simulink model "form_control"  (R2021a)
settings: Solver=VariableStepAuto  StartTime=0.0  StopTime=10.0  RelTol=1e-3
values from neighbouring files (symbols this model uses):
  altitude_d = 5    [run_swarm.m]
  altitude_i = 0    [run_swarm.m]
  b = fir1(filter_order, cutoff_frequency)    [lowpassfilter.m]    (also in run_swarm.m = 1.14e-07)
  g = 9.81    [run_swarm.m]
  I_xx = 4.856e-3    (= 0.004856)    [run_swarm.m]
  I_yy = 4.856e-3    (= 0.004856)    [run_swarm.m]
  I_zz = 8.801e-3    (= 0.008801)    [run_swarm.m]
  Im = 3.357e-5    (= 3.357e-05)    [run_swarm.m]
  k = 2.980e-6    (= 2.98e-06)    [run_swarm.m]
  l = legend(' Leader Position', ' Follower 1 Position','Follower 2 Position','Follower 3 Position')    [Untitled2.m]    (also in run_formation.m; run_swarm.m = legend('$\phi$ Current Y ', '$\phi_d$ Desired Y'); trajVis.m = legend('Desired Trajectory','Actual Trajectory'))
  m = 2    [master_control.m]    (also in run_swarm.m = 0.468)
  pitch_d = -0.1    [run_swarm.m]
  pitch_i = 0    [run_swarm.m]
  roll_d = 0.1    [run_swarm.m]
  roll_i = 0    [run_swarm.m]
  x_i = 0    [run_swarm.m]
  y_i = 0    [run_swarm.m]
  yaw_d = 0.3    [run_swarm.m]
  yaw_i = 0    [run_swarm.m]
libraries: slpidlib x4
settings Model: Creator=templ  LastModifiedBy=templ
settings SolverCC: ZeroCrossAlgorithm=Adaptive
settings DataIOCC: ReturnWorkspaceOutputs=off
settings DebuggingCC: IgnoredZcDiagnostic=none

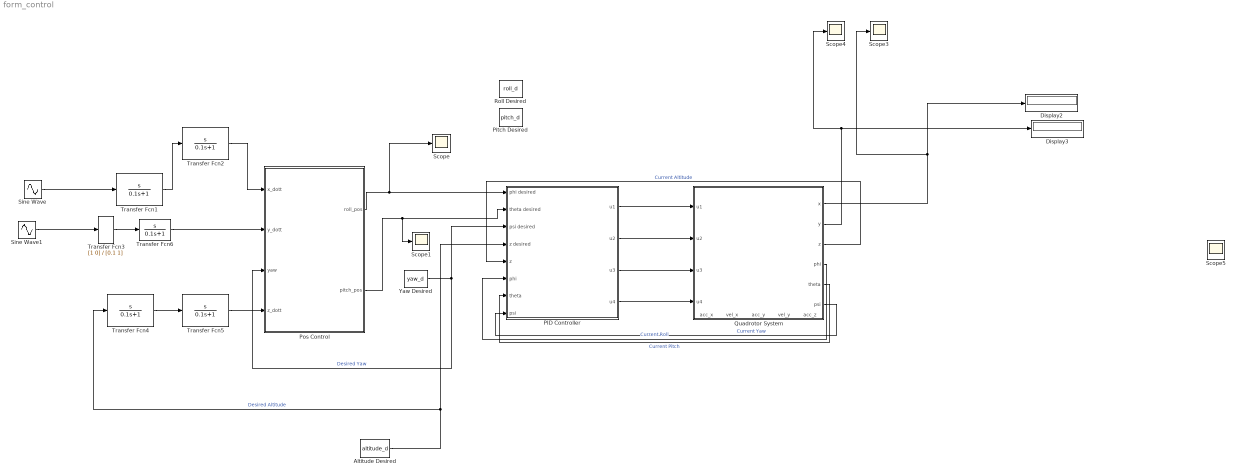
== system form_control ==
  Altitude Desired : Constant  Value=altitude_d
  Display2 : Display
  Display3 : Display
  PID Controller : Subsystem
  Pitch Desired : Constant  Value=pitch_d
  Pos Control : Subsystem
  Quadrotor System : Subsystem
      settings: PortSchema="{\"entries\":[{\"content\":{\"sides\":[{\"content\":{\"connectorIds\":[\"In1\",\"In2\",\"In3\",\"In4\"]},\"type\":\"ConnectorPlacement.EquallySpacedRectSide\",\"uuid\":\"996ed3cc-9aaf-410e-b93a-635ba5fc3cd9\"},{\"content\":{\"connectorIds\":[\"Out1\",\"Out2\",\"Out3\",\"Out4\",\"Out5\",\"Out6\"],\"side\":\"RIGHT\"},\"type\":\"ConnectorPlacement.EquallySpacedRectSide\",\"uuid\":\"7f76db3a-2ef6-433f-bd76-6f00d3bb4716\"},{\"content\":{\"connectorIds\":[],\"side\":\"TOP\"},\"type\":\"ConnectorPlacement.EquallySpacedRectSide\",\"uuid\":\"aa5fab1b-1d66-4c7a-823f-11c675c2f3d7\"},{\"content\":{\"connectorIds\":[\"Out7\",\"Out8\",\"Out9\",\"Out10\",\"Out11\"],\"side\":\"BOTTOM\"},\"type\":\"ConnectorPlacement.EquallySpacedRectSide\",\"uuid\":\"3e671b71-6d8e-4eea-a1dc-38ca984631fc\"}]},\"type\":\"ConnectorPlacement.EquallySpacedConnector\",\"uuid\":\"affe78d5-0f1f-4e1a-8cab-0d93ed3cb974\"}],\"packageUris\":[\"http://schema.mathworks.com/mf0/Connector/R2020b\"],\"version\":\"1.0\"}"
      mask Display: image('C:\Users\angel\OneDrive - Universidad Politécnica de Yucatán\CIMAT\1st semester\Robotic Systems Modeling and Control\Project\Quadrotor\images\quadrotor.jpg');
  Roll Desired : Constant  Value=roll_d
  Scope{,1,3..5} (5 alike) : Scope
  Sine Wave : Sin  SampleTime=0
  Sine Wave1 : Sin  SampleTime=0
  Transfer Fcn{1..6} (6 alike) : TransferFcn  Numerator=[1 0]  Denominator=[0.1 1]
  Yaw Desired : Constant  Value=yaw_d
  wires:
  Quadrotor System/1(x) -> Scope3/1, Display2/1
  Quadrotor System/3(z) -> PID Controller/5(z)  "Current Altitude"
  Quadrotor System/2(y) -> Scope4/1, Display3/1
  Quadrotor System/5(theta) -> PID Controller/7(theta)  "Current Pitch"
  Quadrotor System/4(phi) -> PID Controller/6(phi)  "Current Roll"
  Altitude Desired/1 -> Transfer Fcn4/1, PID Controller/4(z desired)  "Desired Altitude"
  Yaw Desired/1 -> PID Controller/3(psi desired), Pos Control/3(yaw)  "Desired Yaw"
  PID Controller/3(u3) -> Quadrotor System/3(u3)
  PID Controller/4(u4) -> Quadrotor System/4(u4)
  PID Controller/2(u2) -> Quadrotor System/2(u2)
  Quadrotor System/6(psi) -> PID Controller/8(psi)  "Current Yaw"
  PID Controller/1(u1) -> Quadrotor System/1(u1)
  Transfer Fcn2/1 -> Pos Control/1(x_dott)
  Sine Wave/1 -> Transfer Fcn1/1
  Sine Wave1/1 -> Transfer Fcn3/1
  Transfer Fcn6/1 -> Pos Control/2(y_dott)
  Pos Control/1(roll_pos) -> Scope/1, PID Controller/1(phi desired)
  Pos Control/2(pitch_pos) -> Scope1/1, PID Controller/2(theta desired)
  Transfer Fcn5/1 -> Pos Control/4(z_dott)
  Transfer Fcn4/1 -> Transfer Fcn5/1
  Transfer Fcn1/1 -> Transfer Fcn2/1
  Transfer Fcn3/1 -> Transfer Fcn6/1

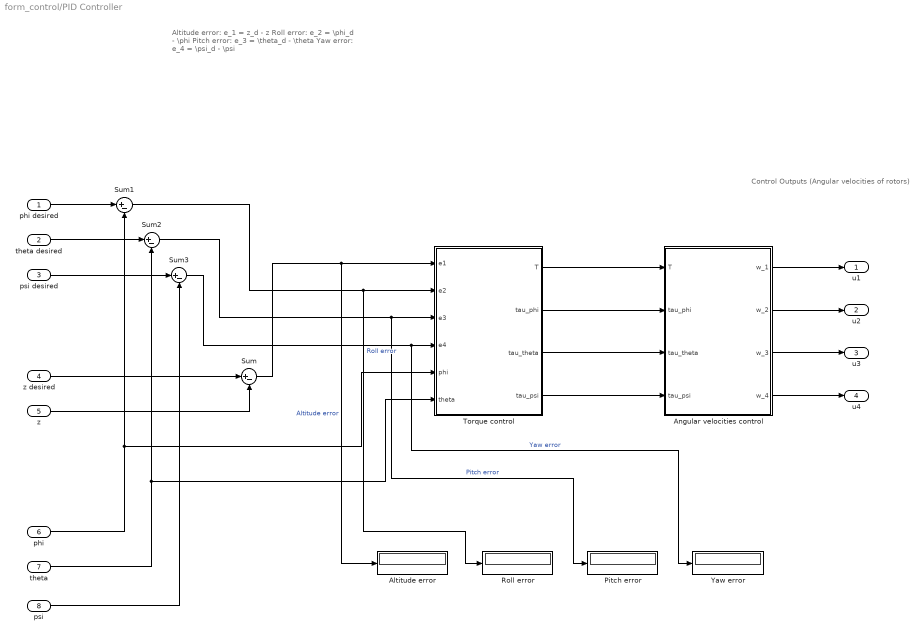
== system form_control/PID Controller ==
  note: Control Outputs
      | (Angular velocities of rotors)
  note: Altitude error: e_1 = z_d - z
      | Roll error: e_2 = \phi_d - \phi
      | Pitch error: e_3 = \theta_d - \theta
      | Yaw error: e_4 = \psi_d - \psi
  phi desired : Inport
  theta desired : Inport  Port=2
  psi desired : Inport  Port=3
  z desired : Inport  Port=4
  z : Inport  Port=5
  phi : Inport  Port=6
  theta : Inport  Port=7
  psi : Inport  Port=8
  Altitude error : Display
  Angular velocities control : Subsystem
  Pitch error : Display
  Roll error : Display
  Sum{,1..3} (4 alike) : Sum  Inputs=|+-
  Torque control : Subsystem
  Yaw error : Display
  u1 : Outport
  u2 : Outport  Port=2
  u3 : Outport  Port=3
  u4 : Outport  Port=4
  wires:
  z desired/1 -> Sum/1
  z/1 -> Sum/2
  Sum/1 -> Altitude error/1, Torque control/1(e1)  "Altitude error"
  phi desired/1 -> Sum1/1
  phi/1 -> Torque control/5("phi "), Sum1/2
  theta desired/1 -> Sum2/1
  theta/1 -> Sum2/2, Torque control/6("theta ")
  psi desired/1 -> Sum3/1
  psi/1 -> Sum3/2
  Sum1/1 -> Roll error/1, Torque control/2(e2)  "Roll error"
  Sum2/1 -> Pitch error/1, Torque control/3(e3)  "Pitch error"
  Sum3/1 -> Yaw error/1, Torque control/4(e4)  "Yaw error"
  Torque control/1(T) -> Angular velocities control/1(T)
  Torque control/2(tau_phi) -> Angular velocities control/2(tau_phi)
  Torque control/3(tau_theta) -> Angular velocities control/3(tau_theta)
  Torque control/4(tau_psi) -> Angular velocities control/4("tau_psi ")
  Angular velocities control/1(w_1) -> u1/1
  Angular velocities control/2(w_2) -> u2/1
  Angular velocities control/3(w_3) -> u3/1
  Angular velocities control/4("w_4 ") -> u4/1

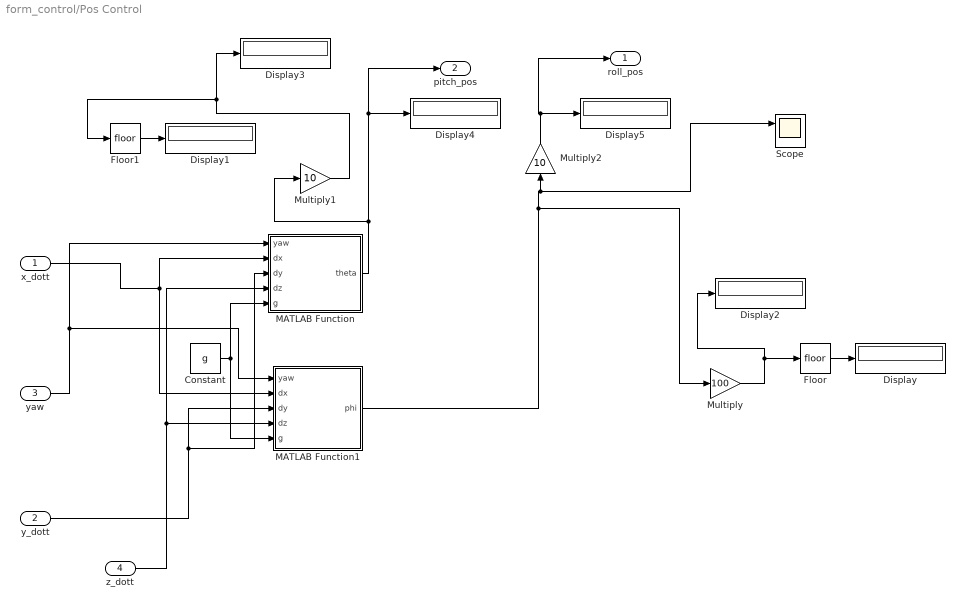
== system form_control/Pos Control ==
  x_dott : Inport
  y_dott : Inport  Port=2
  yaw : Inport  Port=3
  z_dott : Inport  Port=4
  Constant : Constant  Value=g
  Display{,1..5} (6 alike) : Display
  Floor : Rounding
  Floor1 : Rounding
  MATLAB Function : MATLAB Function  TreatAsAtomicUnit=on
  MATLAB Function1 : MATLAB Function  TreatAsAtomicUnit=on
  Multiply : Gain  Gain=100
  Multiply1 : Gain  Gain=10
  Multiply2 : Gain  Gain=10
  Scope : Scope  NumInputPorts=2
  roll_pos : Outport
  pitch_pos : Outport  Port=2
  wires:
  yaw/1 -> MATLAB Function/1(yaw), MATLAB Function1/1(yaw)
  Constant/1 -> MATLAB Function/5(g), MATLAB Function1/5(g)
  MATLAB Function1/1(phi) -> Multiply2/1, Scope/1, Multiply/1
  x_dott/1 -> MATLAB Function1/2(dx), MATLAB Function/2(dx)
  y_dott/1 -> MATLAB Function/3(dy), MATLAB Function1/3(dy)
  Multiply/1 -> Display2/1, Floor/1
  z_dott/1 -> MATLAB Function1/4(dz), MATLAB Function/4(dz)
  MATLAB Function/1(theta) -> pitch_pos/1, Display4/1, Multiply1/1
  Floor/1 -> Display/1
  Multiply1/1 -> Display3/1, Floor1/1
  Floor1/1 -> Display1/1
  Multiply2/1 -> roll_pos/1, Display5/1

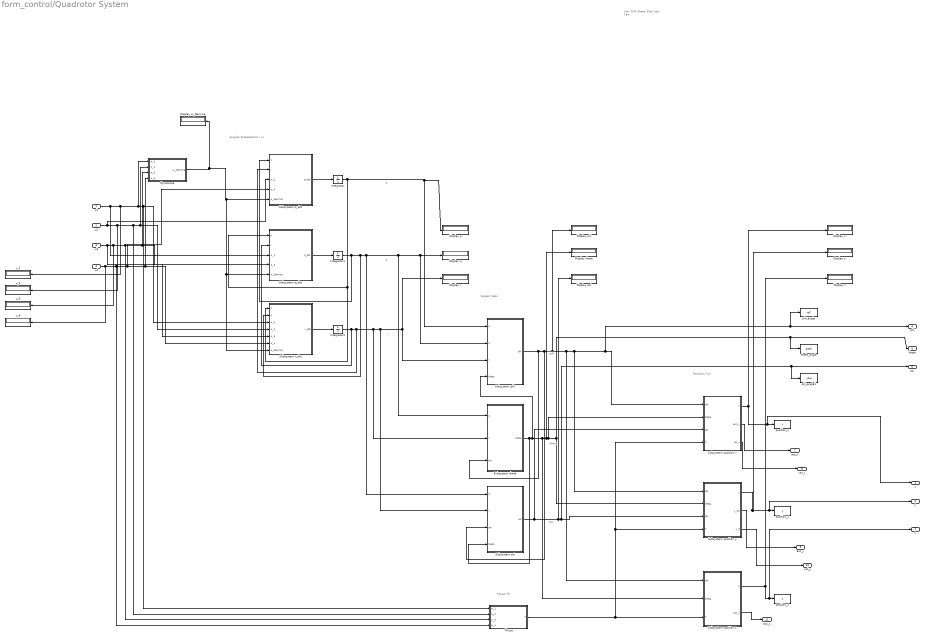
== system form_control/Quadrotor System ==
  note: Angular Accelerations (\nu)
  note: .
  note: \phi: Roll
      | \theta: Pitch
      | \psi: Yaw
  note: Positions (\xi)
  note: Angles (\eta)
  note: Thrust (T)
  note: p
  note: q
  note: r
  note: \phi
  note: \theta
  note: \psi
  u1 : Inport
  u2 : Inport  Port=2
  u3 : Inport  Port=3
  u4 : Inport  Port=4
  Display p : Display
  Display phi : Display
  Display psi : Display
  Display q : Display
  Display r : Display
  Display theta : Display
  Display w_Gamma : Display
  Display x : Display
  Display y : Display
  Display z : Display
  Gyroscope : MATLAB Function  TreatAsAtomicUnit=on
  Integrator : Integrator
  Integrator1 : Integrator
  Integrator2 : Integrator
  Subsystem p_dot : Subsystem
  Subsystem phi : Subsystem
  Subsystem position x : Subsystem
  Subsystem position y : Subsystem
  Subsystem position z : Subsystem
  Subsystem psi : Subsystem
  Subsystem q_dot : Subsystem
  Subsystem r_dot : Subsystem
  Subsystem theta : Subsystem
  Thrust : MATLAB Function  TreatAsAtomicUnit=on
  phi_angle : ToWorkspace  VariableName=roll  SampleTime=-1
  phi_angle1 : ToWorkspace  VariableName=yaw  SampleTime=-1
  position_x : ToWorkspace  VariableName=x  SampleTime=-1
  position_y : ToWorkspace  VariableName=y  SampleTime=-1
  position_z : ToWorkspace  VariableName=z  SampleTime=-1
  theta_angle : ToWorkspace  VariableName=pitch  SampleTime=-1
  u_{1..4} (4 alike) : Display
  x : Outport
  y : Outport  Port=2
  z : Outport  Port=3
  phi : Outport  Port=4
  theta : Outport  Port=5
  psi : Outport  Port=6
  acc_x : Outport  Port=7
  vel_x : Outport  Port=8
  acc_y : Outport  Port=9
  vel_y : Outport  Port=10
  acc_z : Outport  Port=11
  wires:
  u1/1 -> Subsystem q_dot/3(w_1), u_1/1, Gyroscope/1(w_1), Subsystem r_dot/3(w_1), Thrust/1(w_1)
  u2/1 -> Subsystem p_dot/3(w_2), u_2/1, Gyroscope/2(w_2), Subsystem r_dot/4(w_2), Thrust/2(w_2)
  u3/1 -> Subsystem q_dot/4(w_3), Gyroscope/3(w_3), Subsystem r_dot/5(w_3), Thrust/3(w_3), u_3/1
  u4/1 -> u_4/1, Gyroscope/4(w_4), Subsystem r_dot/6(w_4), Subsystem p_dot/4(w_4), Thrust/4(w_4)
  Thrust/1(T) -> Subsystem position y/4("T "), Subsystem position x/4(T), Subsystem position z/3(T)
  Subsystem phi/1("phi ") -> Subsystem theta/3("phi "), Subsystem psi/3(phi), Display phi/1, Subsystem position z/1("phi "), Subsystem position y/1("phi "), phi_angle/1, phi/1, Subsystem position x/1("phi ")
  Subsystem psi/1(psi) -> Subsystem position x/3("psi "), Display psi/1, phi_angle1/1, psi/1, Subsystem position y/3("psi ")
  Subsystem position x/1(x) -> x/1, position_x/1, Display x/1
  Subsystem position z/1(z) -> z/1, position_z/1, Display z/1
  Subsystem position y/1("y ") -> Display y/1, y/1, position_y/1
  Gyroscope/1(w_Gamma) -> Display w_Gamma/1, Subsystem r_dot/7(w_Gamma), Subsystem q_dot/5("w_Gamma "), Subsystem p_dot/5("w_Gamma ")
  Subsystem p_dot/1(p_dot) -> Integrator/1
  Subsystem q_dot/1(q_dot) -> Integrator1/1
  Subsystem r_dot/1(r_dot) -> Integrator2/1
  Integrator/1 -> Subsystem r_dot/1("p "), Subsystem q_dot/1("p "), Display p/1, Subsystem phi/1(p)
  Integrator2/1 -> Subsystem theta/2(r), Subsystem psi/2(r), Display r/1, Subsystem phi/3(r), Subsystem p_dot/2(r), Subsystem q_dot/2(r)
  Integrator1/1 -> Subsystem p_dot/1(q), Subsystem psi/1(q), Subsystem theta/1(q), Display q/1, Subsystem phi/2(q), Subsystem r_dot/2(q)
  Subsystem theta/1(theta) -> Subsystem psi/4(theta), Subsystem phi/4(theta), Subsystem position z/2("theta "), Display theta/1, Subsystem position x/2("theta "), theta_angle/1, theta/1, Subsystem position y/2("theta ")
  Subsystem position x/2(acc_x) -> acc_x/1
  Subsystem position x/3(vel_x) -> vel_x/1
  Subsystem position y/2(y_dd) -> acc_y/1
  Subsystem position y/3(y_d) -> vel_y/1
  Subsystem position z/2(acc_z) -> acc_z/1

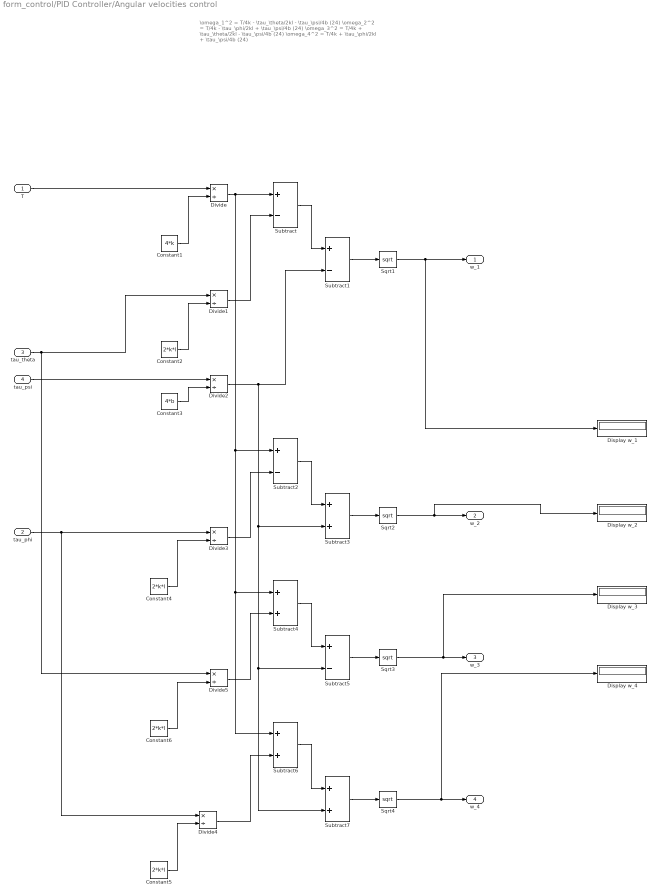
== system form_control/PID Controller/Angular velocities control ==
  note: \omega_1^2 = T/4k - \tau_\theta/2kl - \tau_\psi/4b   (24)
      |
      | \omega_2^2 = T/4k - \tau_\phi/2kl + \tau_\psi/4b   (24)
      |
      | \omega_3^2 = T/4k + \tau_\theta/2kl - \tau_\psi/4b   (24)
      |
      | \omega_4^2 = T/4k + \tau_\phi/2kl + \tau_\psi/4b   (24)
  T : Inport
  tau_phi : Inport  Port=2
  tau_theta : Inport  Port=3
  "tau_psi " : Inport  Port=4
  Constant1 : Constant  Value=4*k
  Constant{2,4..6} (4 alike) : Constant  Value=2*k*l
  Constant3 : Constant  Value=4*b
  Display w_{1..4} (4 alike) : Display
  Divide{,1..5} (6 alike) : Product  Inputs=*/
  Sqrt{1..4} (4 alike) : Sqrt  OutputSignalType=real  SaturateOnIntegerOverflow=on
  Subtract{,1..2,5} (4 alike) : Sum  Inputs=+-
  Subtract{3..4,6..7} (4 alike) : Sum
  w_1 : Outport
  w_2 : Outport  Port=2
  w_3 : Outport  Port=3
  "w_4 " : Outport  Port=4
  wires:
  Constant1/1 -> Divide/2
  T/1 -> Divide/1
  Divide/1 -> Subtract4/1, Subtract6/1, Subtract2/1, Subtract/1
  Constant2/1 -> Divide1/2
  tau_theta/1 -> Divide5/1, Divide1/1
  Divide1/1 -> Subtract/2
  Subtract/1 -> Subtract1/1
  Constant3/1 -> Divide2/2
  Subtract1/1 -> Sqrt1/1
  Sqrt1/1 -> Display w_1/1, w_1/1
  Constant4/1 -> Divide3/2
  tau_phi/1 -> Divide4/1, Divide3/1
  Divide3/1 -> Subtract2/2
  Subtract2/1 -> Subtract3/1
  "tau_psi "/1 -> Divide2/1
  Divide2/1 -> Subtract7/2, Subtract5/2, Subtract3/2, Subtract1/2
  Sqrt2/1 -> Display w_2/1, w_2/1
  Subtract3/1 -> Sqrt2/1
  Constant6/1 -> Divide5/2
  Divide5/1 -> Subtract4/2
  Subtract5/1 -> Sqrt3/1
  Subtract4/1 -> Subtract5/1
  Sqrt3/1 -> Display w_3/1, w_3/1
  Subtract7/1 -> Sqrt4/1
  Constant5/1 -> Divide4/2
  Divide4/1 -> Subtract6/2
  Subtract6/1 -> Subtract7/1
  Sqrt4/1 -> Display w_4/1, "w_4 "/1

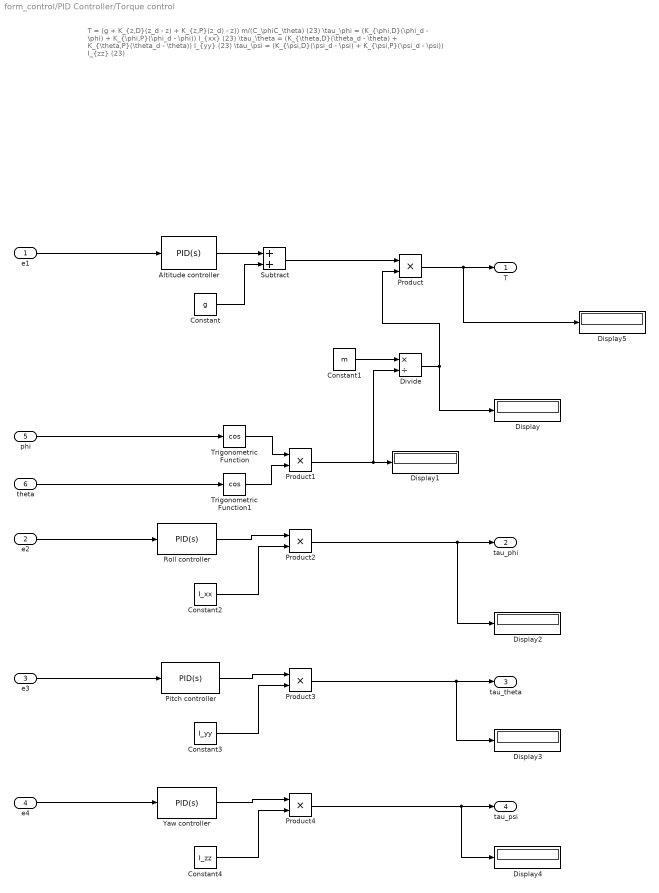
== system form_control/PID Controller/Torque control ==
  note: T = (g + K_{z,D}(z_d - z) + K_{z,P}(z_d) - z)) m/(C_\phiC_\theta)     (23)
      |
      | \tau_\phi = (K_{\phi,D}(\phi_d - \phi) + K_{\phi,P}(\phi_d - \phi)) I_{xx}                   (23)
      |
      | \tau_\theta = (K_{\theta,D}(\theta_d - \theta) + K_{\theta,P}(\theta_d - \theta)) I_{yy}                    (23)
      |
      | \tau_\psi = (K_{\psi,D}(\psi_d - \psi) + K_{\psi,P}(\psi_d - \psi)) I_{zz}                (23)
  e1 : Inport
  e2 : Inport  Port=2
  e3 : Inport  Port=3
  e4 : Inport  Port=4
  "phi " : Inport  Port=5
  "theta " : Inport  Port=6
  Altitude controller : slpidlib/PID Controller  Controller=PID  Form=Parallel  TimeDomain=Continuous-time  UseExternalTs=off  SampleTime=-1  IntegratorMethod=Forward Euler  FilterMethod=Forward Euler  ControllerParametersSource=internal  P=57  I=0.001  D=23  UseFilter=on  N=572.770791824146  TunerSelectOption=Transfer Function Based (PID Tuner App)  InitialConditionSource=internal  InitialConditionForIntegrator=0  InitialConditionForFilter=0  DifferentiatorICPrevScaledInput=0  ExternalReset=none  TrackingMode=off  Kt=1  LimitOutput=on  SatLimitsSource=internal  UpperSaturationLimit=5  LowerSaturationLimit=-5  LinearizeAsGain=on  AntiWindupMode=none  Kb=1  POutMin=[]  POutMax=[]  IOutMin=[]  IOutMax=[]  DOutMin=[]  DOutMax=[]  NOutMin=[]  NOutMax=[]  SumOutMin=[]  SumOutMax=[]  SaturationOutMin=[]  SaturationOutMax=[]  PParamMin=[]  PParamMax=[]  IParamMin=[]  IParamMax=[]  DParamMin=[]  DParamMax=[]  NParamMin=[]  NParamMax=[]  KbParamMin=[]  KbParamMax=[]  KtParamMin=[]  KtParamMax=[]  KbOutMin=[]  KbOutMax=[]  KtOutMin=[]  KtOutMax=[]  IntegratorOutMin=[]  IntegratorOutMax=[]  FilterOutMin=[]  FilterOutMax=[]  SumI1OutMin=[]  SumI1OutMax=[]  SumI2OutMin=[]  SumI2OutMax=[]  SumI3OutMin=[]  SumI3OutMax=[]  SumI4OutMin=[]  SumI4OutMax=[]  SumDOutMin=[]  SumDOutMax=[]  DifferentiatorOutMin=[]  DifferentiatorOutMax=[]  FilterDiffOutCoefMin=[]  FilterDiffOutCoefMax=[]  ReciprocalOutMin=[]  ReciprocalOutMax=[]  SumDenOutMin=[]  SumDenOutMax=[]  SumNumOutMin=[]  SumNumOutMax=[]  DivideOutMin=[]  DivideOutMax=[]  UdiffTsProdOutMin=[]  UdiffTsProdOutMax=[]  NTsProdOutMin=[]  NTsProdOutMax=[]  UintegralTsProdOutMin=[]  UintegralTsProdOutMax=[]  UngainTsProdOutMin=[]  UngainTsProdOutMax=[]  IntegratorContinuousStateAttributes=''  IntegratorStateMustResolveToSignalObject=off  IntegratorRTWStateStorageClass=Auto  FilterContinuousStateAttributes=''  FilterStateMustResolveToSignalObject=off  FilterRTWStateStorageClass=Auto  ParallelPVariant=InternalParameters  IdealPVariant=Disabled  IVariant=InternalParameters  DVariant=InternalParameters  IntegratorVariant=Continuous  SatVariant=Enabled  AWVariant=Passthrough  PCopyVariant=Disabled  TRVariant=Disabled  FdbkBlocksVariant=Forward  IdealPFdbkVariant=Disabled  SatFdbkVariant=Disabled  DerivativeFilterVariant=ContFilter  NVariant=InternalParameters  NCopyVariant=Disabled  FilterICVariant=InternalICsFilter  IntegratorICVariant=InternalICs  ExternalResetVariant=Disabled  TRSumVariant=Passthrough  SumFdbkVariant=Disabled  SumVariant=Sum_PID  TsampFilterVariant=InternalTs  TsampNgainVariant=Passthrough  TsampIntegralVariant=Passthrough  ExternalSaturationOutDataTypeStr=Inherit: Same as second input
  Constant : Constant  Value=g
  Constant1 : Constant  Value=m
  Constant2 : Constant  Value=I_xx
  Constant3 : Constant  Value=I_yy
  Constant4 : Constant  Value=I_zz
  Display{,1..5} (6 alike) : Display
  Divide : Product  Inputs=*/
  Pitch controller : slpidlib/PID Controller  Controller=PID  Form=Parallel  TimeDomain=Continuous-time  UseExternalTs=off  SampleTime=-1  IntegratorMethod=Forward Euler  FilterMethod=Forward Euler  ControllerParametersSource=internal  P=55  I=0.01  D=11  UseFilter=on  N=1414.64809761679  TunerSelectOption=Transfer Function Based (PID Tuner App)  InitialConditionSource=internal  InitialConditionForIntegrator=0  InitialConditionForFilter=0  DifferentiatorICPrevScaledInput=0  ExternalReset=none  TrackingMode=off  Kt=1  LimitOutput=on  SatLimitsSource=internal  UpperSaturationLimit=0.9  LowerSaturationLimit=-0.9  LinearizeAsGain=on  AntiWindupMode=none  Kb=1  POutMin=[]  POutMax=[]  IOutMin=[]  IOutMax=[]  DOutMin=[]  DOutMax=[]  NOutMin=[]  NOutMax=[]  SumOutMin=[]  SumOutMax=[]  SaturationOutMin=[]  SaturationOutMax=[]  PParamMin=[]  PParamMax=[]  IParamMin=[]  IParamMax=[]  DParamMin=[]  DParamMax=[]  NParamMin=[]  NParamMax=[]  KbParamMin=[]  KbParamMax=[]  KtParamMin=[]  KtParamMax=[]  KbOutMin=[]  KbOutMax=[]  KtOutMin=[]  KtOutMax=[]  IntegratorOutMin=[]  IntegratorOutMax=[]  FilterOutMin=[]  FilterOutMax=[]  SumI1OutMin=[]  SumI1OutMax=[]  SumI2OutMin=[]  SumI2OutMax=[]  SumI3OutMin=[]  SumI3OutMax=[]  SumI4OutMin=[]  SumI4OutMax=[]  SumDOutMin=[]  SumDOutMax=[]  DifferentiatorOutMin=[]  DifferentiatorOutMax=[]  FilterDiffOutCoefMin=[]  FilterDiffOutCoefMax=[]  ReciprocalOutMin=[]  ReciprocalOutMax=[]  SumDenOutMin=[]  SumDenOutMax=[]  SumNumOutMin=[]  SumNumOutMax=[]  DivideOutMin=[]  DivideOutMax=[]  UdiffTsProdOutMin=[]  UdiffTsProdOutMax=[]  NTsProdOutMin=[]  NTsProdOutMax=[]  UintegralTsProdOutMin=[]  UintegralTsProdOutMax=[]  UngainTsProdOutMin=[]  UngainTsProdOutMax=[]  IntegratorContinuousStateAttributes=''  IntegratorStateMustResolveToSignalObject=off  IntegratorRTWStateStorageClass=Auto  FilterContinuousStateAttributes=''  FilterStateMustResolveToSignalObject=off  FilterRTWStateStorageClass=Auto  ParallelPVariant=InternalParameters  IdealPVariant=Disabled  IVariant=InternalParameters  DVariant=InternalParameters  IntegratorVariant=Continuous  SatVariant=Enabled  AWVariant=Passthrough  PCopyVariant=Disabled  TRVariant=Disabled  FdbkBlocksVariant=Forward  IdealPFdbkVariant=Disabled  SatFdbkVariant=Disabled  DerivativeFilterVariant=ContFilter  NVariant=InternalParameters  NCopyVariant=Disabled  FilterICVariant=InternalICsFilter  IntegratorICVariant=InternalICs  ExternalResetVariant=Disabled  TRSumVariant=Passthrough  SumFdbkVariant=Disabled  SumVariant=Sum_PID  TsampFilterVariant=InternalTs  TsampNgainVariant=Passthrough  TsampIntegralVariant=Passthrough  ExternalSaturationOutDataTypeStr=Inherit: Same as second input
  Product{,1..4} (5 alike) : Product
  Roll controller : slpidlib/PID Controller  Controller=PID  Form=Parallel  TimeDomain=Continuous-time  UseExternalTs=off  SampleTime=-1  IntegratorMethod=Forward Euler  FilterMethod=Forward Euler  ControllerParametersSource=internal  P=55  I=0.01  D=18  UseFilter=on  N=1414.64809761679  TunerSelectOption=Transfer Function Based (PID Tuner App)  InitialConditionSource=internal  InitialConditionForIntegrator=0  InitialConditionForFilter=0  DifferentiatorICPrevScaledInput=0  ExternalReset=none  TrackingMode=off  Kt=1  LimitOutput=on  SatLimitsSource=internal  UpperSaturationLimit=0.9  LowerSaturationLimit=-0.9  LinearizeAsGain=on  AntiWindupMode=none  Kb=1  POutMin=[]  POutMax=[]  IOutMin=[]  IOutMax=[]  DOutMin=[]  DOutMax=[]  NOutMin=[]  NOutMax=[]  SumOutMin=[]  SumOutMax=[]  SaturationOutMin=[]  SaturationOutMax=[]  PParamMin=[]  PParamMax=[]  IParamMin=[]  IParamMax=[]  DParamMin=[]  DParamMax=[]  NParamMin=[]  NParamMax=[]  KbParamMin=[]  KbParamMax=[]  KtParamMin=[]  KtParamMax=[]  KbOutMin=[]  KbOutMax=[]  KtOutMin=[]  KtOutMax=[]  IntegratorOutMin=[]  IntegratorOutMax=[]  FilterOutMin=[]  FilterOutMax=[]  SumI1OutMin=[]  SumI1OutMax=[]  SumI2OutMin=[]  SumI2OutMax=[]  SumI3OutMin=[]  SumI3OutMax=[]  SumI4OutMin=[]  SumI4OutMax=[]  SumDOutMin=[]  SumDOutMax=[]  DifferentiatorOutMin=[]  DifferentiatorOutMax=[]  FilterDiffOutCoefMin=[]  FilterDiffOutCoefMax=[]  ReciprocalOutMin=[]  ReciprocalOutMax=[]  SumDenOutMin=[]  SumDenOutMax=[]  SumNumOutMin=[]  SumNumOutMax=[]  DivideOutMin=[]  DivideOutMax=[]  UdiffTsProdOutMin=[]  UdiffTsProdOutMax=[]  NTsProdOutMin=[]  NTsProdOutMax=[]  UintegralTsProdOutMin=[]  UintegralTsProdOutMax=[]  UngainTsProdOutMin=[]  UngainTsProdOutMax=[]  IntegratorContinuousStateAttributes=''  IntegratorStateMustResolveToSignalObject=off  IntegratorRTWStateStorageClass=Auto  FilterContinuousStateAttributes=''  FilterStateMustResolveToSignalObject=off  FilterRTWStateStorageClass=Auto  ParallelPVariant=InternalParameters  IdealPVariant=Disabled  IVariant=InternalParameters  DVariant=InternalParameters  IntegratorVariant=Continuous  SatVariant=Enabled  AWVariant=Passthrough  PCopyVariant=Disabled  TRVariant=Disabled  FdbkBlocksVariant=Forward  IdealPFdbkVariant=Disabled  SatFdbkVariant=Disabled  DerivativeFilterVariant=ContFilter  NVariant=InternalParameters  NCopyVariant=Disabled  FilterICVariant=InternalICsFilter  IntegratorICVariant=InternalICs  ExternalResetVariant=Disabled  TRSumVariant=Passthrough  SumFdbkVariant=Disabled  SumVariant=Sum_PID  TsampFilterVariant=InternalTs  TsampNgainVariant=Passthrough  TsampIntegralVariant=Passthrough  ExternalSaturationOutDataTypeStr=Inherit: Same as second input
  Subtract : Sum
  Trigonometric Function : Trigonometry  Operator=cos
  Trigonometric Function1 : Trigonometry  Operator=cos
  Yaw controller : slpidlib/PID Controller  Controller=PID  Form=Parallel  TimeDomain=Continuous-time  UseExternalTs=off  SampleTime=-1  IntegratorMethod=Forward Euler  FilterMethod=Forward Euler  ControllerParametersSource=internal  P=53  I=0.04  D=26.2  UseFilter=on  N=95.667343116538  TunerSelectOption=Transfer Function Based (PID Tuner App)  InitialConditionSource=internal  InitialConditionForIntegrator=0  InitialConditionForFilter=0  DifferentiatorICPrevScaledInput=0  ExternalReset=none  TrackingMode=off  Kt=1  LimitOutput=on  SatLimitsSource=internal  UpperSaturationLimit=5  LowerSaturationLimit=-5  LinearizeAsGain=on  AntiWindupMode=none  Kb=1  POutMin=[]  POutMax=[]  IOutMin=[]  IOutMax=[]  DOutMin=[]  DOutMax=[]  NOutMin=[]  NOutMax=[]  SumOutMin=[]  SumOutMax=[]  SaturationOutMin=[]  SaturationOutMax=[]  PParamMin=[]  PParamMax=[]  IParamMin=[]  IParamMax=[]  DParamMin=[]  DParamMax=[]  NParamMin=[]  NParamMax=[]  KbParamMin=[]  KbParamMax=[]  KtParamMin=[]  KtParamMax=[]  KbOutMin=[]  KbOutMax=[]  KtOutMin=[]  KtOutMax=[]  IntegratorOutMin=[]  IntegratorOutMax=[]  FilterOutMin=[]  FilterOutMax=[]  SumI1OutMin=[]  SumI1OutMax=[]  SumI2OutMin=[]  SumI2OutMax=[]  SumI3OutMin=[]  SumI3OutMax=[]  SumI4OutMin=[]  SumI4OutMax=[]  SumDOutMin=[]  SumDOutMax=[]  DifferentiatorOutMin=[]  DifferentiatorOutMax=[]  FilterDiffOutCoefMin=[]  FilterDiffOutCoefMax=[]  ReciprocalOutMin=[]  ReciprocalOutMax=[]  SumDenOutMin=[]  SumDenOutMax=[]  SumNumOutMin=[]  SumNumOutMax=[]  DivideOutMin=[]  DivideOutMax=[]  UdiffTsProdOutMin=[]  UdiffTsProdOutMax=[]  NTsProdOutMin=[]  NTsProdOutMax=[]  UintegralTsProdOutMin=[]  UintegralTsProdOutMax=[]  UngainTsProdOutMin=[]  UngainTsProdOutMax=[]  IntegratorContinuousStateAttributes=''  IntegratorStateMustResolveToSignalObject=off  IntegratorRTWStateStorageClass=Auto  FilterContinuousStateAttributes=''  FilterStateMustResolveToSignalObject=off  FilterRTWStateStorageClass=Auto  ParallelPVariant=InternalParameters  IdealPVariant=Disabled  IVariant=InternalParameters  DVariant=InternalParameters  IntegratorVariant=Continuous  SatVariant=Enabled  AWVariant=Passthrough  PCopyVariant=Disabled  TRVariant=Disabled  FdbkBlocksVariant=Forward  IdealPFdbkVariant=Disabled  SatFdbkVariant=Disabled  DerivativeFilterVariant=ContFilter  NVariant=InternalParameters  NCopyVariant=Disabled  FilterICVariant=InternalICsFilter  IntegratorICVariant=InternalICs  ExternalResetVariant=Disabled  TRSumVariant=Passthrough  SumFdbkVariant=Disabled  SumVariant=Sum_PID  TsampFilterVariant=InternalTs  TsampNgainVariant=Passthrough  TsampIntegralVariant=Passthrough  ExternalSaturationOutDataTypeStr=Inherit: Same as second input
  T : Outport
  tau_phi : Outport  Port=2
  tau_theta : Outport  Port=3
  tau_psi : Outport  Port=4
  wires:
  Constant/1 -> Subtract/2
  e1/1 -> Altitude controller/1
  Altitude controller/1 -> Subtract/1
  Subtract/1 -> Product/1
  Constant1/1 -> Divide/1
  Divide/1 -> Product/2, Display/1
  "phi "/1 -> Trigonometric Function/1
  "theta "/1 -> Trigonometric Function1/1
  Trigonometric Function/1 -> Product1/1
  Trigonometric Function1/1 -> Product1/2
  Product1/1 -> Display1/1, Divide/2
  Product/1 -> Display5/1, T/1
  e2/1 -> Roll controller/1
  Roll controller/1 -> Product2/1
  Constant2/1 -> Product2/2
  Product2/1 -> Display2/1, tau_phi/1
  Constant3/1 -> Product3/2
  Pitch controller/1 -> Product3/1
  Constant4/1 -> Product4/2
  Yaw controller/1 -> Product4/1
  e4/1 -> Yaw controller/1
  e3/1 -> Pitch controller/1
  Product3/1 -> Display3/1, tau_theta/1
  Product4/1 -> Display4/1, tau_psi/1

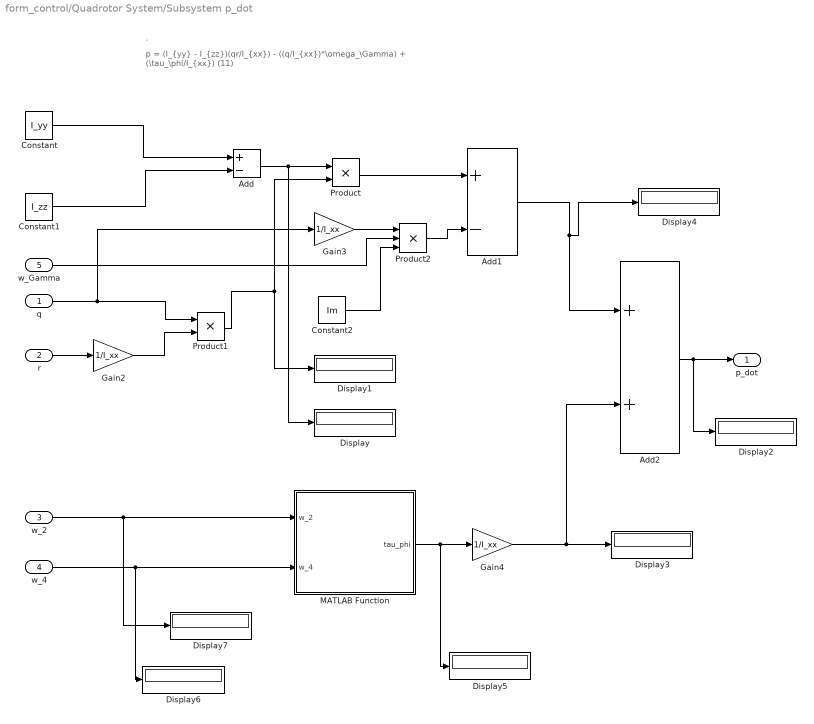
== system form_control/Quadrotor System/Subsystem p_dot ==
  note: p = (I_{yy} - I_{zz})(qr/I_{xx}) - ((q/I_{xx})*\omega_\Gamma) + (\tau_\phi/I_{xx}) (11)
  note: .
  q : Inport
  r : Inport  Port=2
  w_2 : Inport  Port=3
  w_4 : Inport  Port=4
  "w_Gamma " : Inport  Port=5
  Add : Sum  Inputs=+-
  Add1 : Sum  Inputs=+-
  Add2 : Sum
  Constant : Constant  Value=I_yy
  Constant1 : Constant  Value=I_zz
  Constant2 : Constant  Value=Im
  Display{,1..7} (8 alike) : Display
  Gain2 : Gain  Gain=1/I_xx
  Gain3 : Gain  Gain=1/I_xx
  Gain4 : Gain  Gain=1/I_xx
  MATLAB Function : MATLAB Function  TreatAsAtomicUnit=on
  Product : Product
  Product1 : Product
  Product2 : Product  Inputs=3
  p_dot : Outport
  wires:
  Constant/1 -> Add/1
  Constant1/1 -> Add/2
  Add/1 -> Display/1, Product/1
  Product/1 -> Add1/1
  Product2/1 -> Add1/2
  Add2/1 -> p_dot/1, Display2/1
  r/1 -> Gain2/1
  Gain2/1 -> Product1/2
  q/1 -> Gain3/1, Product1/1
  Gain3/1 -> Product2/1
  Product1/1 -> Display1/1, Product/2
  MATLAB Function/1(tau_phi) -> Display5/1, Gain4/1
  w_2/1 -> MATLAB Function/1(w_2), Display7/1
  w_4/1 -> Display6/1, MATLAB Function/2(w_4)
  "w_Gamma "/1 -> Product2/2
  Gain4/1 -> Display3/1, Add2/2
  Add1/1 -> Display4/1, Add2/1
  Constant2/1 -> Product2/3

== system form_control/Quadrotor System/Subsystem phi ==
  note: \phi
  note: \phi
  note: .
  note: \phi = p + q(S_\phiT_\theta) + r(C_\phiT_\theta) (4)
  note: .
  p : Inport
  q : Inport  Port=2
  r : Inport  Port=3
  theta : Inport  Port=4
  Display1 : Display
  Display10 : Display
  Display9 : Display
  Integrator6 : Integrator  InitialConditionSource=external  InitialCondition=-0.1
  Product5 : Product  Inputs=3
  Product6 : Product  Inputs=3
  Roll Initial : Constant  Value=roll_i
  Z''3 : Sum  Inputs=+++
  "cos " : Trigonometry  Operator=cos
  cos 1 : Trigonometry
  tan 1 : Trigonometry  Operator=tan
  tan 5 : Trigonometry  Operator=tan
  "phi " : Outport
  wires:
  "cos "/1 -> Product5/1
  Product5/1 -> Display10/1, Z''3/1
  theta/1 -> tan 5/1, tan 1/1
  Integrator6/1 -> "cos "/1, Display1/1, cos 1/1, "phi "/1
  tan 5/1 -> Product5/3
  Z''3/1 -> Integrator6/1
  q/1 -> Product6/2
  Product6/1 -> Display9/1, Z''3/3
  p/1 -> Z''3/2
  cos 1/1 -> Product6/1
  tan 1/1 -> Product6/3
  r/1 -> Product5/2
  Roll Initial/1 -> Integrator6/2

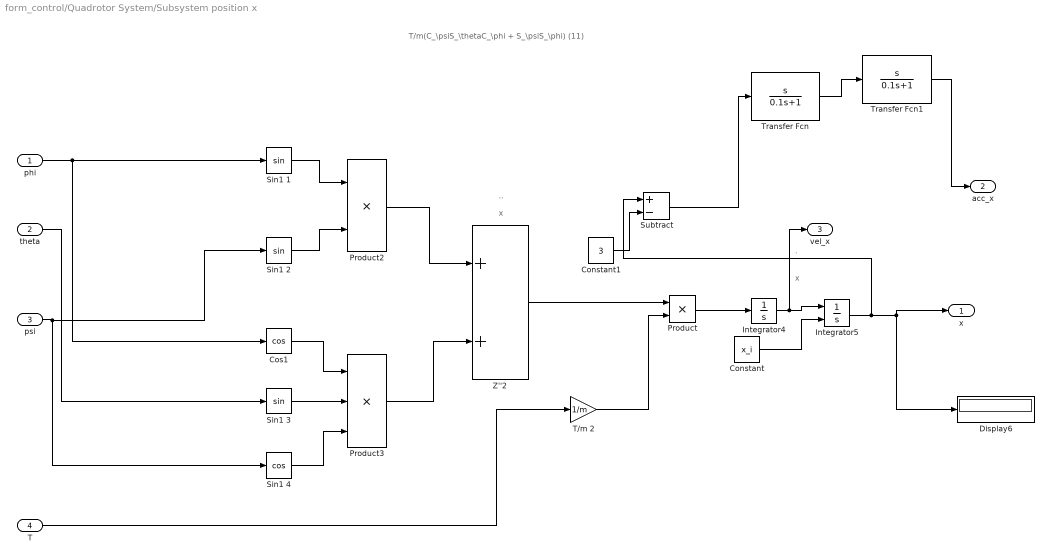
== system form_control/Quadrotor System/Subsystem position x ==
  note: ..
  note: x
  note: .
  note: x
  note: T/m(C_\psiS_\thetaC_\phi + S_\psiS_\phi) (11)
  "phi " : Inport
  "theta " : Inport  Port=2
  "psi " : Inport  Port=3
  T : Inport  Port=4
  Constant : Constant  Value=x_i
  Constant1 : Constant  Value=3
  Cos1 : Trigonometry  Operator=cos
  Display6 : Display
  Integrator4 : Integrator
  Integrator5 : Integrator  InitialConditionSource=external
  Product : Product
  Product2 : Product
  Product3 : Product  Inputs=3
  Sin1 1 : Trigonometry
  Sin1 2 : Trigonometry
  Sin1 3 : Trigonometry
  Sin1 4 : Trigonometry  Operator=cos
  Subtract : Sum  Inputs=+-
  T/m 2 : Gain  Gain=1/m
  Transfer Fcn : TransferFcn  Numerator=[1 0]  Denominator=[0.1 1]
  Transfer Fcn1 : TransferFcn  Numerator=[1 0]  Denominator=[0.1 1]
  Z''2 : Sum
  x : Outport
  acc_x : Outport  Port=2
  vel_x : Outport  Port=3
  wires:
  "phi "/1 -> Cos1/1, Sin1 1/1
  "psi "/1 -> Sin1 2/1, Sin1 4/1
  Integrator4/1 -> vel_x/1, Integrator5/1
  Product2/1 -> Z''2/1
  Product3/1 -> Z''2/2
  "theta "/1 -> Sin1 3/1
  Sin1 1/1 -> Product2/1
  Sin1 3/1 -> Product3/2
  Sin1 2/1 -> Product2/2
  Sin1 4/1 -> Product3/3
  Cos1/1 -> Product3/1
  Integrator5/1 -> Subtract/1, x/1, Display6/1
  T/m 2/1 -> Product/2
  T/1 -> T/m 2/1
  Z''2/1 -> Product/1
  Constant/1 -> Integrator5/2
  Product/1 -> Integrator4/1
  Constant1/1 -> Subtract/2
  Transfer Fcn/1 -> Transfer Fcn1/1
  Transfer Fcn1/1 -> acc_x/1
  Subtract/1 -> Transfer Fcn/1

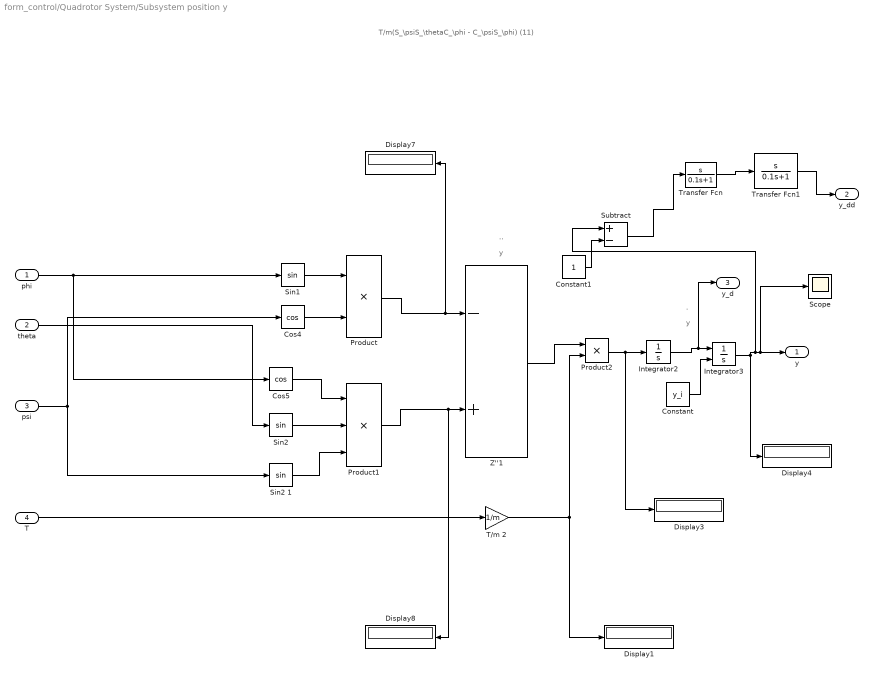
== system form_control/Quadrotor System/Subsystem position y ==
  note: T/m(S_\psiS_\thetaC_\phi - C_\psiS_\phi) (11)
  note: ..
  note: y
  note: y
  note: .
  "phi " : Inport
  "theta " : Inport  Port=2
  "psi " : Inport  Port=3
  "T " : Inport  Port=4
  Constant : Constant  Value=y_i
  Constant1 : Constant
  Cos4 : Trigonometry  Operator=cos
  Cos5 : Trigonometry  Operator=cos
  Display{1,3..4,7..8} (5 alike) : Display
  Integrator2 : Integrator
  Integrator3 : Integrator  InitialConditionSource=external
  Product : Product
  Product1 : Product  Inputs=3
  Product2 : Product
  Scope : Scope
  "Sin1 " : Trigonometry
  "Sin2 " : Trigonometry
  Sin2 1 : Trigonometry
  Subtract : Sum  Inputs=+-
  T/m 2 : Gain  Gain=1/m
  Transfer Fcn : TransferFcn  Numerator=[1 0]  Denominator=[0.1 1]
  Transfer Fcn1 : TransferFcn  Numerator=[1 0]  Denominator=[0.1 1]
  Z''1 : Sum  Inputs=-+
  "y " : Outport
  y_dd : Outport  Port=2
  y_d : Outport  Port=3
  wires:
  Integrator2/1 -> y_d/1, Integrator3/1
  "theta "/1 -> "Sin2 "/1
  Integrator3/1 -> Subtract/1, "y "/1, Scope/1, Display4/1
  "phi "/1 -> "Sin1 "/1, Cos5/1
  Product/1 -> Display7/1, Z''1/1
  Cos4/1 -> Product/2
  "psi "/1 -> Cos4/1, Sin2 1/1
  Sin2 1/1 -> Product1/3
  Product1/1 -> Display8/1, Z''1/2
  Cos5/1 -> Product1/1
  "Sin2 "/1 -> Product1/2
  "Sin1 "/1 -> Product/1
  "T "/1 -> T/m 2/1
  Z''1/1 -> Product2/1
  T/m 2/1 -> Display1/1, Product2/2
  Constant/1 -> Integrator3/2
  Product2/1 -> Display3/1, Integrator2/1
  Constant1/1 -> Subtract/2
  Transfer Fcn1/1 -> y_dd/1
  Transfer Fcn/1 -> Transfer Fcn1/1
  Subtract/1 -> Transfer Fcn/1

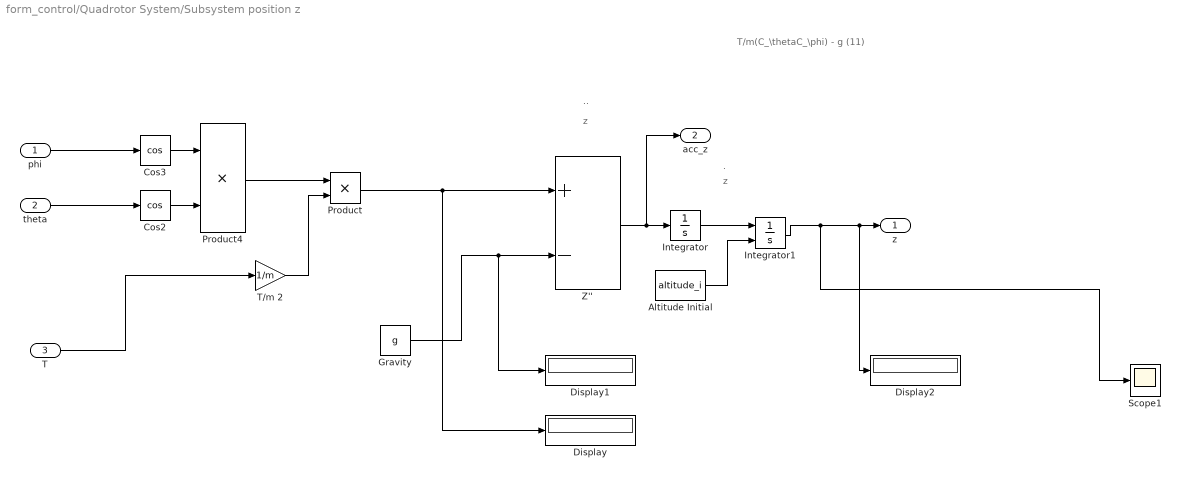
== system form_control/Quadrotor System/Subsystem position z ==
  note: z
  note: ..
  note: .
  note: z
  note: T/m(C_\thetaC_\phi) - g (11)
  "phi " : Inport
  "theta " : Inport  Port=2
  T : Inport  Port=3
  Altitude Initial : Constant  Value=altitude_i
  Cos2 : Trigonometry  Operator=cos
  Cos3 : Trigonometry  Operator=cos
  Display : Display
  Display1 : Display
  Display2 : Display
  Gravity : Constant  Value=g
  Integrator : Integrator
  Integrator1 : Integrator  InitialConditionSource=external
  Product : Product
  Product4 : Product
  Scope1 : Scope
  T/m 2 : Gain  Gain=1/m
  Z'' : Sum  Inputs=+-
  z : Outport
  acc_z : Outport  Port=2
  wires:
  "phi "/1 -> Cos3/1
  Gravity/1 -> Display1/1, Z''/2
  Z''/1 -> acc_z/1, Integrator/1
  Integrator1/1 -> z/1, Display2/1, Scope1/1
  "theta "/1 -> Cos2/1
  Integrator/1 -> Integrator1/1
  Cos2/1 -> Product4/2
  Cos3/1 -> Product4/1
  T/1 -> T/m 2/1
  Product4/1 -> Product/1
  Product/1 -> Display/1, Z''/1
  T/m 2/1 -> Product/2
  Altitude Initial/1 -> Integrator1/2

== system form_control/Quadrotor System/Subsystem psi ==
  note: .
  note: \psi
  note: \psi
  note: \psi = q(S_\phi/C_\theta) + r(C_\phi/C_\theta) (4)
  note: .
  q : Inport
  r : Inport  Port=2
  phi : Inport  Port=3
  theta : Inport  Port=4
  Display1 : Display
  Display16 : Display
  Display17 : Display
  Divide : Product  Inputs=/
  Divide1 : Product  Inputs=/
  Integrator8 : Integrator  InitialConditionSource=external  InitialCondition=-pi
  Product10 : Product  Inputs=3
  Product9 : Product  Inputs=3
  Yaw Initial : Constant  Value=yaw_i
  Z''5 : Sum
  sin 3 : Trigonometry  Operator=cos
  sin 4 : Trigonometry  Operator=cos
  sin 5 : Trigonometry
  sin 6 : Trigonometry  Operator=cos
  psi : Outport
  wires:
  sin 3/1 -> Product9/1
  Divide1/1 -> Product10/3
  sin 5/1 -> Product10/1
  sin 4/1 -> Divide/1
  Divide/1 -> Product9/3
  sin 6/1 -> Divide1/1
  Product9/1 -> Display16/1, Z''5/1
  theta/1 -> sin 6/1, sin 4/1
  phi/1 -> sin 5/1, sin 3/1
  q/1 -> Product10/2
  r/1 -> Product9/2
  Z''5/1 -> Integrator8/1
  Product10/1 -> Display17/1, Z''5/2
  Integrator8/1 -> Display1/1, psi/1
  Yaw Initial/1 -> Integrator8/2

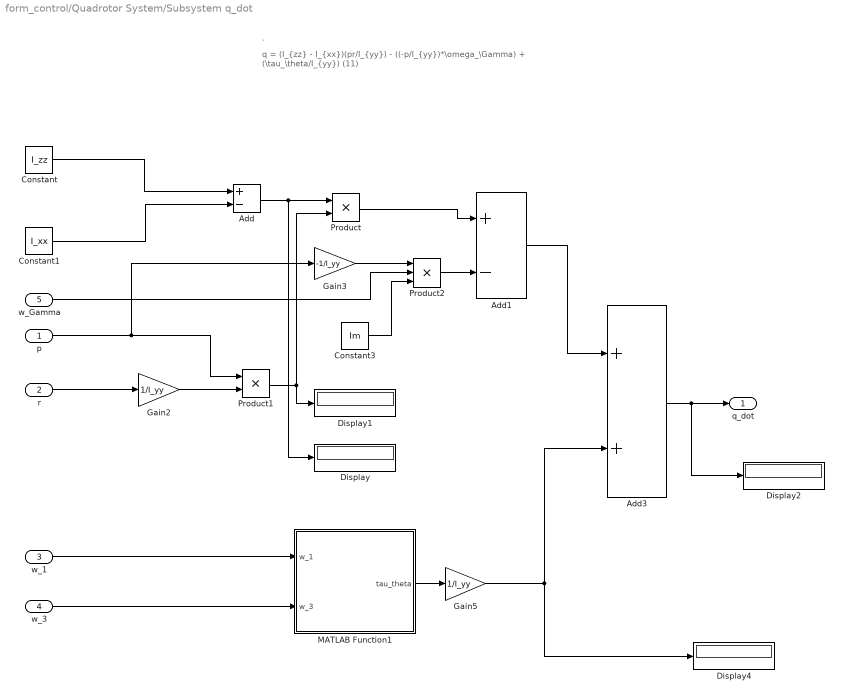
== system form_control/Quadrotor System/Subsystem q_dot ==
  note: q = (I_{zz} - I_{xx})(pr/I_{yy}) - ((-p/I_{yy})*\omega_\Gamma) + (\tau_\theta/I_{yy}) (11)
  note: .
  "p " : Inport
  r : Inport  Port=2
  w_1 : Inport  Port=3
  w_3 : Inport  Port=4
  "w_Gamma " : Inport  Port=5
  Add : Sum  Inputs=+-
  Add1 : Sum  Inputs=+-
  Add3 : Sum
  Constant : Constant  Value=I_zz
  Constant1 : Constant  Value=I_xx
  Constant3 : Constant  Value=Im
  Display{,1..2,4} (4 alike) : Display
  Gain2 : Gain  Gain=1/I_yy
  Gain3 : Gain  Gain=-1/I_yy
  Gain5 : Gain  Gain=1/I_yy
  MATLAB Function1 : MATLAB Function  TreatAsAtomicUnit=on
  Product : Product
  Product1 : Product
  Product2 : Product  Inputs=3
  q_dot : Outport
  wires:
  Constant/1 -> Add/1
  Constant1/1 -> Add/2
  Add/1 -> Display/1, Product/1
  Product1/1 -> Product/2, Display1/1
  Product/1 -> Add1/1
  Gain3/1 -> Product2/1
  Product2/1 -> Add1/2
  r/1 -> Gain2/1
  Gain2/1 -> Product1/2
  "p "/1 -> Gain3/1, Product1/1
  w_3/1 -> MATLAB Function1/2(w_3)
  MATLAB Function1/1(tau_theta) -> Gain5/1
  w_1/1 -> MATLAB Function1/1(w_1)
  Add1/1 -> Add3/1
  Add3/1 -> q_dot/1, Display2/1
  "w_Gamma "/1 -> Product2/2
  Gain5/1 -> Display4/1, Add3/2
  Constant3/1 -> Product2/3

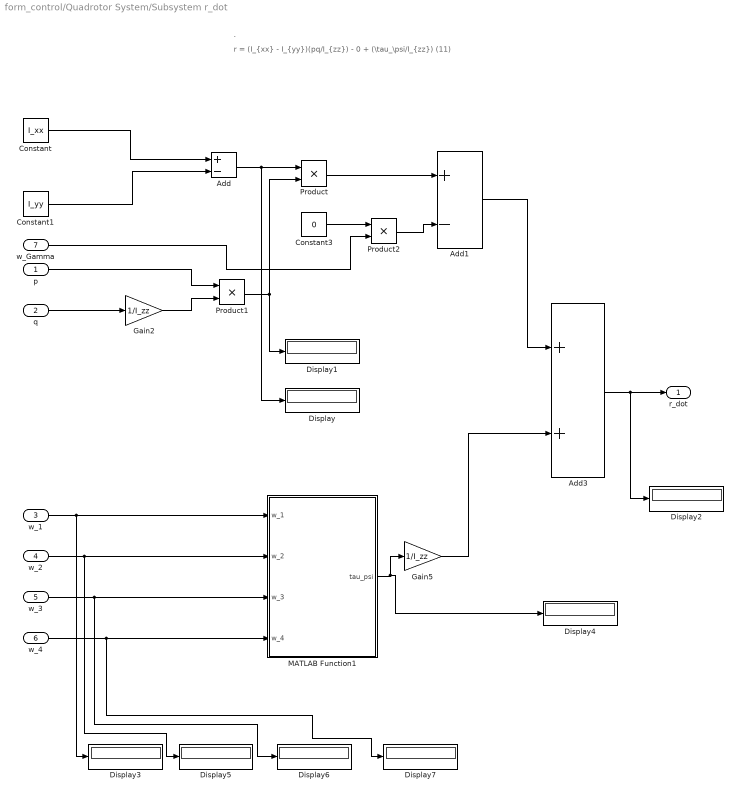
== system form_control/Quadrotor System/Subsystem r_dot ==
  note: r = (I_{xx} - I_{yy})(pq/I_{zz}) - 0 + (\tau_\psi/I_{zz}) (11)
  note: .
  "p " : Inport
  q : Inport  Port=2
  w_1 : Inport  Port=3
  w_2 : Inport  Port=4
  w_3 : Inport  Port=5
  w_4 : Inport  Port=6
  w_Gamma : Inport  Port=7
  Add : Sum  Inputs=+-
  Add1 : Sum  Inputs=+-
  Add3 : Sum
  Constant : Constant  Value=I_xx
  Constant1 : Constant  Value=I_yy
  Constant3 : Constant  Value=0
  Display{,1..7} (8 alike) : Display
  Gain2 : Gain  Gain=1/I_zz
  Gain5 : Gain  Gain=1/I_zz
  MATLAB Function1 : MATLAB Function  TreatAsAtomicUnit=on
  Product : Product
  Product1 : Product
  Product2 : Product
  r_dot : Outport
  wires:
  Constant/1 -> Add/1
  Constant1/1 -> Add/2
  Add/1 -> Display/1, Product/1
  Product1/1 -> Display1/1, Product/2
  Product/1 -> Add1/1
  Constant3/1 -> Product2/1
  Product2/1 -> Add1/2
  Add1/1 -> Add3/1
  Add3/1 -> Display2/1, r_dot/1
  "p "/1 -> Product1/1
  Gain2/1 -> Product1/2
  q/1 -> Gain2/1
  MATLAB Function1/1(tau_psi) -> Display4/1, Gain5/1
  w_1/1 -> MATLAB Function1/1(w_1), Display3/1
  w_2/1 -> MATLAB Function1/2(w_2), Display5/1
  w_4/1 -> MATLAB Function1/4(w_4), Display7/1
  w_Gamma/1 -> Product2/2
  Gain5/1 -> Add3/2
  w_3/1 -> MATLAB Function1/3(w_3), Display6/1

== system form_control/Quadrotor System/Subsystem theta ==
  note: \theta
  note: .
  note: \theta
  note: .
  note: \theta = q(C_\phi) - r(S_\theta) (4)
  q : Inport
  r : Inport  Port=2
  "phi " : Inport  Port=3
  Display1 : Display
  Display13 : Display
  Display14 : Display
  Integrator7 : Integrator  InitialConditionSource=external  InitialCondition=-0.09
  Pitch Initial : Constant  Value=pitch_i
  Product7 : Product
  Product8 : Product
  Z''4 : Sum  Inputs=-+
  sin 1 : Trigonometry  Operator=cos
  sin 2 : Trigonometry
  theta : Outport
  wires:
  "phi "/1 -> sin 1/1, sin 2/1
  r/1 -> Product7/2
  sin 1/1 -> Product8/1
  Product8/1 -> Display14/1, Z''4/2
  Z''4/1 -> Integrator7/1
  sin 2/1 -> Product7/1
  Product7/1 -> Display13/1, Z''4/1
  q/1 -> Product8/2
  Integrator7/1 -> Display1/1, theta/1
  Pitch Initial/1 -> Integrator7/2

== matlab function form_control/Quadrotor System/Subsystem p_dot/MATLAB Function ==
  data: w_2 input; w_4 input; tau_phi output
function tau_phi = fcn(w_2, w_4)
k = 2.980e-6; % Thrust factor of rotor (depends on density
              % geometry, etc) 
l = 0.225; % Linear distance from the centre of the rotor
           % to the centre of gravity          
tau_phi = l * k * (-w_2^2 + w_4^2);

== matlab function form_control/Quadrotor System/Subsystem q_dot/MATLAB Function1 ==
  data: w_1 input; w_3 input; tau_theta output
function tau_theta = fcn(w_1, w_3)
k = 2.980e-6; % Thrust factor of rotor (depends on density
              % geometry, etc) 
l = 0.225; % Linear distance from the centre of the rotor
           % to the centre of gravity          
tau_theta = l * k * (-w_1^2 + w_3^2);

== matlab function form_control/Quadrotor System/Subsystem r_dot/MATLAB Function1 ==
  data: w_1 input; w_2 input; w_3 input; tau_psi output; w_4 input
function tau_psi = fcn(w_1, w_2, w_3, w_4)
k = 2.980e-6; % Thrust factor of rotor (depends on density
              % geometry, etc) 
l = 0.225; % Linear distance from the centre of the rotor
           % to the centre of gravity    
b = 1.140e-7; % Drag constant
Im = 3.357e-5; % Inertia moment of the rotor
tau_psi = b*(-w_1^2 + w_2^2 - w_3^2 + w_4^2);
% tau_psi = (b * w_1^2 + Im) - (b * w_2^2 + Im) + (b * w_3^2 + Im) - (b * w_4^2 + Im);

== matlab function form_control/Quadrotor System/Gyroscope ==
  data: w_1 input; w_2 input; w_3 input; w_Gamma output; w_4 input
function w_Gamma = fcn(w_1, w_2, w_3, w_4)
    
w_Gamma = w_1 - w_2 + w_3 - w_4;

== matlab function form_control/Quadrotor System/Thrust ==
  data: w_1 input; T output; w_2 input; w_3 input; w_4 input
function T = fcn(w_1, w_2, w_3, w_4)
k = 2.980e-6; % Thrust factor of rotor (depends on density
T = k * (w_1^2 + w_2^2 + w_3^2 + w_4^2);

== matlab function form_control/Pos Control/MATLAB Function ==
  data: yaw input; theta output; dx input; dy input; dz input; g input
function theta = fcn(yaw,dx,dy,dz,g)
buff_pos=(dx*cos(yaw)+dy*sin(yaw))/(g+dz);
%THIS IS PITCH
theta=atan(buff_pos);

end

== matlab function form_control/Pos Control/MATLAB Function1 ==
  data: yaw input; phi output; dx input; dy input; dz input; g input
function phi = fcn(yaw,dx,dy,dz,g)
buff_pos=(dx*sin(yaw)-dy*cos(yaw))/((dx^2)+(dy^2)+(dz+g)^2);
disp(buff_pos)
%THIS IS ROLL
phi=asin((buff_pos));

end
